simulink library "EPBI_lib"  (Simulink 7.5)
settings: Solver=ode45  StartTime=0.0  StopTime=10.0  RelTol=1e-3
libraries: simulink x1
settings Model: Creator=wuaibin  LastModifiedBy=wuaibin

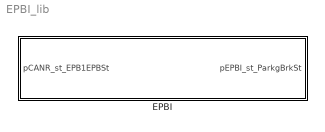
== system EPBI_lib ==
  EPBI : Subsystem  TreatAsAtomicUnit=on

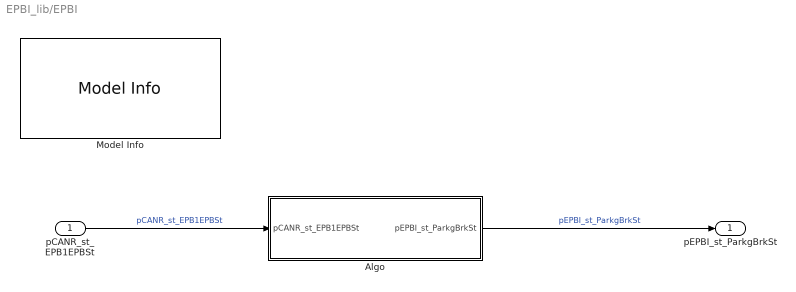
== system EPBI_lib/EPBI ==
  pCANR_st_EPB1EPBSt : Inport  OutDataType=fixdt(1, 16)  OutScaling=2^0
  Algo : Subsystem
  Model Info : simulink/Model-Wide Utilities/Model Info  SystemSampleTime=-1  InitialBlockCM=None  BlockCM=None  Frame=on  DisplayStringWithTags=Model Info\nCreated: %<Created>\nCreator: %<Creator>  HorizontalTextAlignment=Center  LeftAlignmentValue=0.5  SourceBlockDiagram=HQEV_HCU  TagMaxNumber=20
  pEPBI_st_ParkgBrkSt : Outport  OutDataType=fixdt(1, 16)  OutScaling=2^0
  wires:
  pCANR_st_EPB1EPBSt/1 -> Algo/1(pCANR_st_EPB1EPBSt)  "pCANR_st_EPB1EPBSt"
  Algo/1(pEPBI_st_ParkgBrkSt) -> pEPBI_st_ParkgBrkSt/1  "pEPBI_st_ParkgBrkSt"

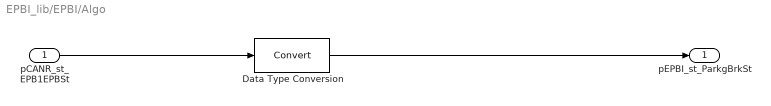
== system EPBI_lib/EPBI/Algo ==
  pCANR_st_EPB1EPBSt : Inport  OutDataType=fixdt(1, 16)  OutScaling=2^0
  Data Type Conversion : DataTypeConversion  OutDataType=fixdt(1, 16)  OutScaling=2^0
  pEPBI_st_ParkgBrkSt : Outport  OutDataType=fixdt(1, 16)  OutScaling=2^0
  wires:
  pCANR_st_EPB1EPBSt/1 -> Data Type Conversion/1
  Data Type Conversion/1 -> pEPBI_st_ParkgBrkSt/1
